simulink model "parallel_decimation_testing2"  (Simulink 7.4)
settings: Solver=ode45  StartTime=0.0  StopTime=100  RelTol=1e-3
libraries: xbsIndex_r4 x49, simulink x2
settings Model: Creator=chenhong  LastModifiedBy=chenhong

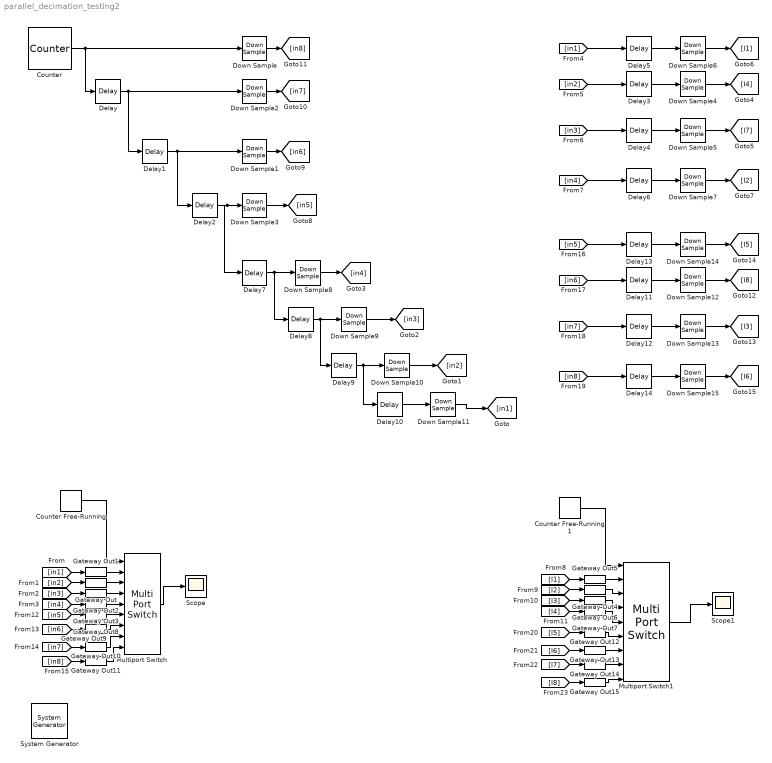
== system parallel_decimation_testing2 ==
  " System Generator" : xbsIndex_r4/ System Generator  Tag=genX  SystemSampleTime=-1  xilinxfamily=Virtex6  part=xc6vsx315t  speed=-3  package=ff1156  synthesis_tool=XST  clock_wrapper=Clock Enables  directory=./netlist  testbench=off  simulink_period=1  sysclk_period=10  dcm_input_clock_period=10  incr_netlist=off  trim_vbits=Everywhere in SubSystem  dbl_ovrd=According to Block Masks  core_generation=According to Block Masks  run_coregen=off  deprecated_control=off  eval_field=0  block_type=sysgen
      settings: block_version=11.4
  Counter : xbsIndex_r4/Counter  cnt_type=Free Running  cnt_to=Inf  operation=Up  start_count=0  cnt_by_val=1  arith_type=Unsigned  n_bits=8  bin_pt=0  load_pin=off  rst=off  en=off  explicit_period=on  period=1  dbl_ovrd=off  use_behavioral_HDL=off  implementation=Fabric  block_type=counter
      settings: block_version=11.4
  Counter Free-Running : simulink/Sources/Counter Free-Running  SystemSampleTime=-1  NumBits=3  tsamp=1
  Counter Free-Running1 : simulink/Sources/Counter Free-Running  SystemSampleTime=-1  NumBits=3  tsamp=3
  Delay{,1..3,7..10,13..14} (10 alike) : xbsIndex_r4/Delay  en=off  latency=1  dbl_ovrd=off  reg_retiming=off  block_type=delay
      settings: block_version=11.4
  Delay11 : xbsIndex_r4/Delay  en=off  latency=0  dbl_ovrd=off  reg_retiming=off  block_type=delay
      settings: block_version=11.4
  Delay12 : xbsIndex_r4/Delay  en=off  latency=2  dbl_ovrd=off  reg_retiming=off  block_type=delay
      settings: block_version=11.4
  Delay4 : xbsIndex_r4/Delay  en=off  latency=0  dbl_ovrd=off  reg_retiming=off  block_type=delay
      settings: block_version=11.4
  Delay5 : xbsIndex_r4/Delay  en=off  latency=2  dbl_ovrd=off  reg_retiming=off  block_type=delay
      settings: block_version=11.4
  Delay6 : xbsIndex_r4/Delay  en=off  latency=2  dbl_ovrd=off  reg_retiming=off  block_type=delay
      settings: block_version=11.4
  Down Sample{,1..3,8..11} (8 alike) : xbsIndex_r4/Down Sample  sample_ratio=8  sample_phase="Last Value of Frame  (most efficient)"  en=off  latency=1  dbl_ovrd=off  block_type=dsamp
      settings: block_version=11.4
  Down Sample{4..7,12..15} (8 alike) : xbsIndex_r4/Down Sample  sample_ratio=3  sample_phase="Last Value of Frame  (most efficient)"  en=off  latency=1  dbl_ovrd=off  block_type=dsamp
      settings: block_version=11.4
  Gateway Out{,1..15} (16 alike) : xbsIndex_r4/Gateway Out  hdl_port=off  timing_constraint=None  locs_specified=off  LOCs={}  block_type=gatewayout
      settings: infoedit="Gateway out block.  Converts Xilinx fixed point inputs into ouputs of type Simulink integer, double, or fixed point.<br><br>Hardware notes:  In hardware these blocks become top level output ports or are discarded, depending on how they are configured."  block_version=11.4
  Multiport Switch : MultiPortSwitch  Inputs=8  zeroidx=on  OutDataType=fixdt(1, 16)  OutScaling=2^0  SampleTime=1
  Multiport Switch1 : MultiPortSwitch  Inputs=8  zeroidx=on  OutDataType=fixdt(1, 16)  OutScaling=2^0  SampleTime=3
  Scope : Scope
  Scope1 : Scope
  wires:
  Counter/1 -> Down Sample/1, Delay/1
  Delay/1 -> Down Sample2/1, Delay1/1
  Delay1/1 -> Down Sample1/1, Delay2/1
  Delay2/1 -> Down Sample3/1, Delay7/1
  Counter Free-Running/1 -> Multiport Switch/1
  Down Sample/1 -> [in8]
  Down Sample2/1 -> [in7]
  Down Sample1/1 -> [in6]
  Down Sample3/1 -> [in5]
  [in1] -> Gateway Out1/1
  [in2] -> Gateway Out/1
  [in3] -> Gateway Out2/1
  [in4] -> Gateway Out3/1
  Gateway Out1/1 -> Multiport Switch/2
  Gateway Out/1 -> Multiport Switch/3
  Gateway Out2/1 -> Multiport Switch/4
  Gateway Out3/1 -> Multiport Switch/5
  Multiport Switch/1 -> Scope/1
  [in2] -> Delay3/1
  Delay3/1 -> Down Sample4/1
  [in3] -> Delay4/1
  Delay4/1 -> Down Sample5/1
  Delay5/1 -> Down Sample6/1
  [in1] -> Delay5/1
  [in4] -> Delay6/1
  Delay6/1 -> Down Sample7/1
  Down Sample4/1 -> [I4]
  Down Sample5/1 -> [I7]
  Down Sample6/1 -> [I1]
  Down Sample7/1 -> [I2]
  Counter Free-Running1/1 -> Multiport Switch1/1
  [I1] -> Gateway Out5/1
  [I2] -> Gateway Out4/1
  [I3] -> Gateway Out6/1
  [I4] -> Gateway Out7/1
  Gateway Out5/1 -> Multiport Switch1/2
  Gateway Out4/1 -> Multiport Switch1/3
  Gateway Out6/1 -> Multiport Switch1/4
  Gateway Out7/1 -> Multiport Switch1/5
  Multiport Switch1/1 -> Scope1/1
  Delay7/1 -> Down Sample8/1, Delay8/1
  Delay8/1 -> Down Sample9/1, Delay9/1
  Delay9/1 -> Down Sample10/1, Delay10/1
  Delay10/1 -> Down Sample11/1
  Down Sample11/1 -> [in1]
  Down Sample10/1 -> [in2]
  Down Sample9/1 -> [in3]
  Down Sample8/1 -> [in4]
  [in5] -> Gateway Out8/1
  Gateway Out8/1 -> Multiport Switch/6
  [in6] -> Gateway Out9/1
  [in7] -> Gateway Out10/1
  [in8] -> Gateway Out11/1
  Gateway Out9/1 -> Multiport Switch/7
  Gateway Out10/1 -> Multiport Switch/8
  Gateway Out11/1 -> Multiport Switch/9
  [in6] -> Delay11/1
  Delay11/1 -> Down Sample12/1
  [in7] -> Delay12/1
  Delay12/1 -> Down Sample13/1
  Delay13/1 -> Down Sample14/1
  [in5] -> Delay13/1
  [in8] -> Delay14/1
  Delay14/1 -> Down Sample15/1
  Down Sample12/1 -> [I8]
  Down Sample13/1 -> [I3]
  Down Sample14/1 -> [I5]
  Down Sample15/1 -> [I6]
  [I5] -> Gateway Out12/1
  [I6] -> Gateway Out13/1
  [I7] -> Gateway Out14/1
  [I8] -> Gateway Out15/1
  Gateway Out12/1 -> Multiport Switch1/6
  Gateway Out13/1 -> Multiport Switch1/7
  Gateway Out14/1 -> Multiport Switch1/8
  Gateway Out15/1 -> Multiport Switch1/9
